simulink model "untitled2"  (Simulink 7.5)
settings: Solver=ode45  StartTime=0.0  StopTime=10.0  RelTol=1e-3
settings Model: Creator=dell  LastModifiedBy=dell

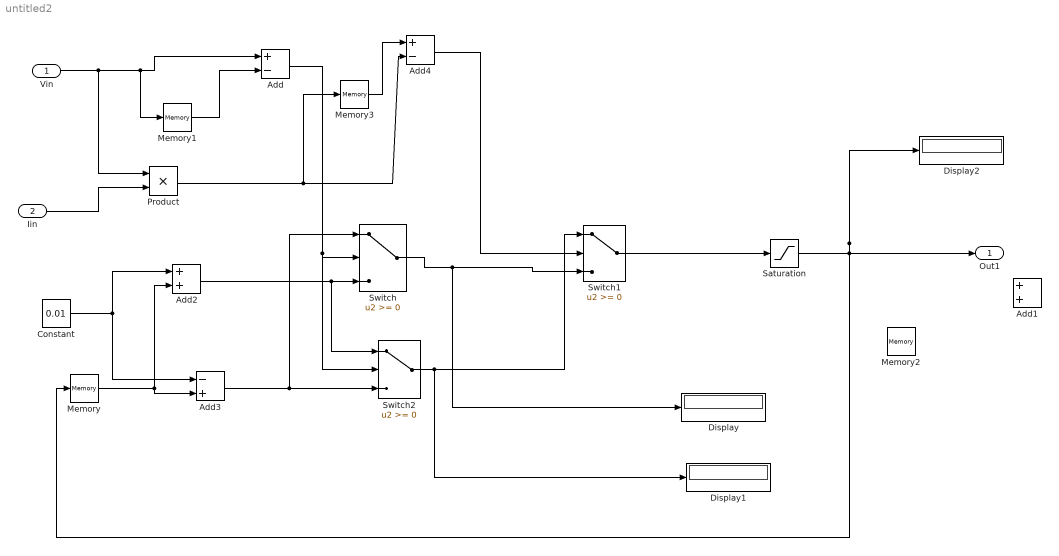
== system untitled2 ==
  Vin : Inport  OutDataType=fixdt(1, 16)  OutScaling=2^0
  Iin : Inport  Port=2  OutDataType=fixdt(1, 16)  OutScaling=2^0
  Add : Sum  Inputs=+-  OutDataType=fixdt(1, 16)  OutScaling=2^-10
  Add1 : Sum  OutDataType=fixdt(1, 16)  OutScaling=2^-10
  Add2 : Sum  OutDataType=fixdt(1, 16)  OutScaling=2^-10
  Add3 : Sum  Inputs=-+  OutDataType=fixdt(1, 16)  OutScaling=2^-10
  Add4 : Sum  Inputs=+-  OutDataType=fixdt(1, 16)  OutScaling=2^-10
  Constant : Constant  Value=0.01  OutDataType=fixdt(1, 16)  OutScaling=2^0
  Display : Display
  Display1 : Display
  Display2 : Display
  Memory{,1..3} (4 alike) : Memory
  Product : Product  OutDataType=fixdt(1, 16)  OutScaling=2^0  RndMeth=Zero
  Saturation : Saturate  OutDataType=fixdt(1, 16)  OutScaling=2^0
  Switch : Switch  OutDataType=fixdt(1, 16)  OutScaling=2^0
  Switch1 : Switch  OutDataType=fixdt(1, 16)  OutScaling=2^0
  Switch2 : Switch  OutDataType=fixdt(1, 16)  OutScaling=2^0
  Out1 : Outport  OutDataType=fixdt(1, 16)  OutScaling=2^0
  wires:
  Vin/1 -> Add/1, Memory1/1, Product/1
  Memory1/1 -> Add/2
  Iin/1 -> Product/2
  Product/1 -> Add4/2, Memory3/1
  Memory3/1 -> Add4/1
  Constant/1 -> Add3/1, Add2/1
  Memory/1 -> Add2/2, Add3/2
  Add2/1 -> Switch/3, Switch2/1
  Add/1 -> Switch/2, Switch2/2
  Add3/1 -> Switch2/3, Switch/1
  Add4/1 -> Switch1/2
  Switch2/1 -> Switch1/1, Display1/1
  Switch/1 -> Switch1/3, Display/1
  Switch1/1 -> Saturation/1
  Saturation/1 -> Display2/1, Memory/1, Out1/1
